simulink model "mdaqdemo_led"  (R2013a)
settings: Solver=FixedStepDiscrete  SolverMode=SingleTasking  StartTime=0.0  StopTime=10.0  FixedStep=0.1  RelTol=1e-3
libraries: simulink x2, microdaq_lib x2
settings Model: Creator=bas  LastModifiedBy=peselnikmg
settings SolverCC: PositivePriorityOrder=on
settings DataIOCC: SaveOutput=off  SaveTime=off
settings OptimizationCC: EnhancedBackFolding=on  OptimizeModelRefInitCode=on  LifeSpan=1
settings HardwareCC: ProdBitPerLong=40  ProdLargestAtomicInteger=Integer  ProdIntDivRoundTo=Zero  ProdEndianess=LittleEndian  ProdHWDeviceType=Texas Instruments->C6000
settings RTWCC: SystemTargetFile=microdaq.tlc  TemplateMakefile=microdaq.tmf  PostCodeGenCommand=microdaq_postcodegen(buildInfo)  Description=MicroDAQ Real-Time Measurement System  GenerateReport=on  ProcessScript=microdaq_make_rtw_hook  IncludeHyperlinkInReport=on  LaunchReport=on  GenerateTraceInfo=on
settings CodeAppCC: IgnoreCustomStorageClasses=off
settings STFCustomTargetCC: CodeReplacementLibrary=TI C674x  CombineOutputUpdateFcns=on  ERTCustomFileBanners=on  SupportContinuousTime=off  SupportNonInlinedSFcns=off  MATLABClassNameForMDSCustomization=Simulink.SoftwareTarget.ERTCustomization  SystemTargetFile=microdaq.tlc
settings ERTTargetCC: CodeReplacementLibrary=TI C674x  GenerateSampleERTMain=off  ParMdlRefBuildCompliant=off  CompOptLevelCompliant=off  ConcurrentExecutionCompliant=off  ERTFirstTimeCompliant=off  ModelStepFunctionPrototypeControlCompliant=off  CPPClassGenCompliant=off  ERTCustomFileTemplate=microdaq_main.tlc

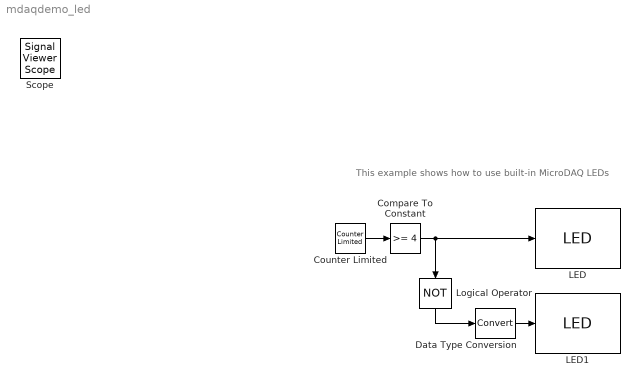
== system mdaqdemo_led ==
  note: This example shows how to use built-in MicroDAQ LEDs
  Compare To Constant : simulink/Logic and Bit Operations/Compare To Constant  relop=>=  const=4  OutDataTypeStr=uint8
  Counter Limited : simulink/Sources/Counter Limited  uplimit=7  tsamp=-1
      settings: AttributesFormatString=Upper limit: %<uplimit>
  Data Type Conversion : DataTypeConversion
  LED : microdaq_lib/LED  SParameter1=D1
      settings: AttributesFormatString=LED: %<SParameter1>
  LED1 : microdaq_lib/LED  SParameter1=D2
      settings: AttributesFormatString=LED: %<SParameter1>
  Logical Operator : Logic  Operator=NOT  AllPortsSameDT=off  OutDataTypeStr=boolean
  Scope : SignalViewerScope  IOType=viewer  RefreshTime=0.035000
  wires:
  Compare To Constant/1 -> Logical Operator/1, LED/1
  Logical Operator/1 -> Data Type Conversion/1
  Data Type Conversion/1 -> LED1/1
  Counter Limited/1 -> Compare To Constant/1
